simulink model "PhaseLockedLoop"  (R2025b)
settings: Solver=VariableStepAuto  StartTime=0.0  StopTime=10  RelTol=1e-3
values from neighbouring files (symbols this model uses):
  fo = 90    [startup.m]
  Ki = 100    [startup.m]
  Kp = 50    [startup.m]
  Kvco = 100    [startup.m]
settings Model: Creator=Chetan  LastModifiedBy=Chetan

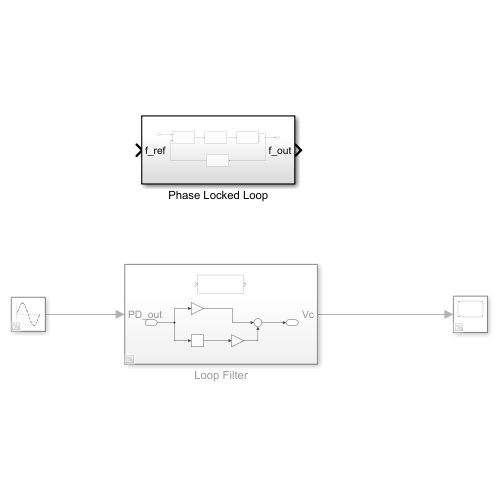
[thumbnail: Simulink's stored preview of the top-level diagram]
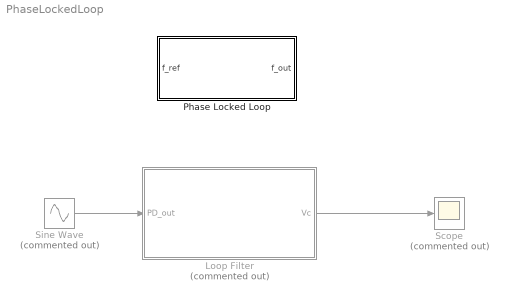
== system PhaseLockedLoop ==
  Loop Filter : Subsystem  Commented=on
  Phase Locked Loop : Subsystem
  Scope : Scope  Commented=on
      settings: ActiveDisplayYMinimum=-36.249999999999993  ActiveDisplayYMaximum=326.25
  Sine Wave : Sin  Commented=on  SampleTime=0
  wires:
  Loop Filter/1(Vc) -> Scope/1
  Sine Wave/1 -> Loop Filter/1(PD_out)

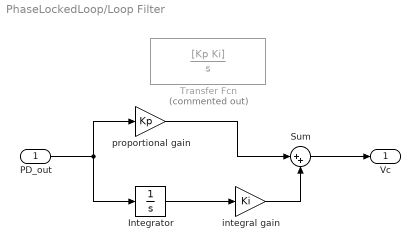
== system PhaseLockedLoop/Loop Filter ==
  PD_out : Inport
  Integrator : Integrator
  Sum : Sum  Inputs=|++
  Transfer Fcn : TransferFcn  Commented=on  Numerator=[Kp Ki]  Denominator=[1 0]  ContinuousStateAttributes='e'
  integral gain : Gain  Gain=Ki
  proportional gain : Gain  Gain=Kp
  Vc : Outport
  wires:
  PD_out/1 -> proportional gain/1, Integrator/1
  Sum/1 -> Vc/1
  Integrator/1 -> integral gain/1
  integral gain/1 -> Sum/2
  proportional gain/1 -> Sum/1

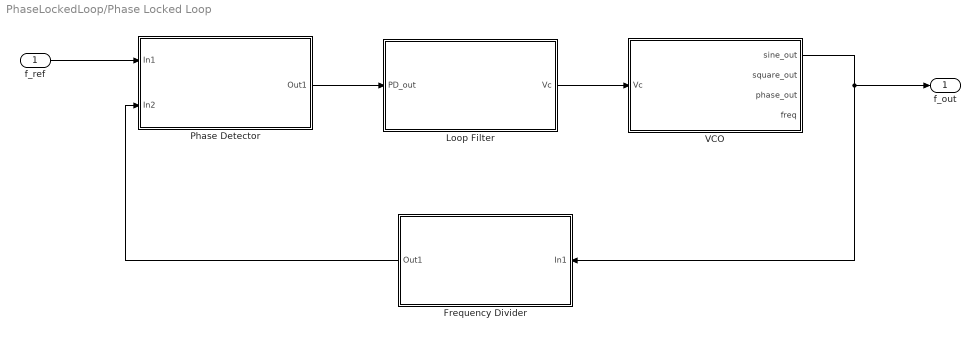
== system PhaseLockedLoop/Phase Locked Loop ==
  f_ref : Inport
  Frequency Divider : Subsystem
  Loop Filter : Subsystem
  Phase Detector : Subsystem
  VCO : Subsystem
  f_out : Outport
  wires:
  Frequency Divider/1(Out1) -> Phase Detector/2(In2)
  VCO/1(sine_out) -> f_out/1, Frequency Divider/1(In1)
  Phase Detector/1(Out1) -> Loop Filter/1(PD_out)
  Loop Filter/1(Vc) -> VCO/1(Vc)
  f_ref/1 -> Phase Detector/1(In1)

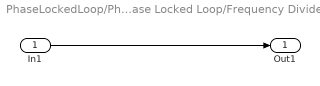
== system PhaseLockedLoop/Phase Locked Loop/Frequency Divider ==
  In1 : Inport
  Out1 : Outport
  wires:
  In1/1 -> Out1/1

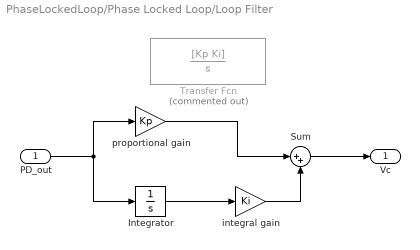
== system PhaseLockedLoop/Phase Locked Loop/Loop Filter ==
  PD_out : Inport
  Integrator : Integrator
  Sum : Sum  Inputs=|++
  Transfer Fcn : TransferFcn  Commented=on  Numerator=[Kp Ki]  Denominator=[1 0]  ContinuousStateAttributes='e'
  integral gain : Gain  Gain=Ki
  proportional gain : Gain  Gain=Kp
  Vc : Outport
  wires:
  PD_out/1 -> proportional gain/1, Integrator/1
  Sum/1 -> Vc/1
  Integrator/1 -> integral gain/1
  integral gain/1 -> Sum/2
  proportional gain/1 -> Sum/1

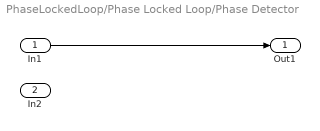
== system PhaseLockedLoop/Phase Locked Loop/Phase Detector ==
  In1 : Inport
  In2 : Inport  Port=2
  Out1 : Outport
  wires:
  In1/1 -> Out1/1

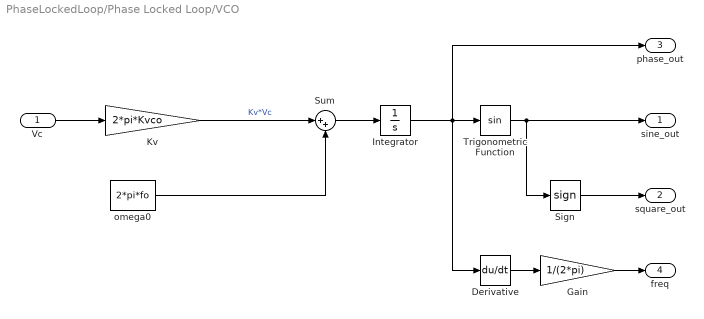
== system PhaseLockedLoop/Phase Locked Loop/VCO ==
  Vc : Inport
  Derivative : Derivative
  Gain : Gain  Gain=1/(2*pi)
  Integrator : Integrator
  Kv : Gain  Gain=2*pi*Kvco
  Sign : Signum
  Sum : Sum  Inputs=|++
  Trigonometric Function : Trigonometry
  omega0 : Constant  Value=2*pi*fo
  sine_out : Outport
  square_out : Outport  Port=2
  phase_out : Outport  Port=3
  freq : Outport  Port=4
  wires:
  Vc/1 -> Kv/1
  Kv/1 -> Sum/1  "Kv*Vc"
  Sum/1 -> Integrator/1
  omega0/1 -> Sum/2
  Integrator/1 -> Derivative/1, phase_out/1, Trigonometric Function/1
  Trigonometric Function/1 -> Sign/1, sine_out/1
  Sign/1 -> square_out/1
  Derivative/1 -> Gain/1
  Gain/1 -> freq/1
